simulink model "Junctions7"  (R2020a)
settings: Solver=FixedStepDiscrete  StartTime=0.0  StopTime=0.1  FixedStep=0.1  RelTol=1e-3  EnableMultiTasking=on
settings Model: Creator=BEAR  LastModifiedBy=bzhan
settings SolverCC: AutoInsertRateTranBlk=on
settings DataIOCC: LimitDataPoints=on  ReturnWorkspaceOutputs=off
settings OptimizationCC: LifeSpan=inf
settings DebuggingCC: AllowSymbolicDim=off  SFUnexpectedBacktrackingDiag=warning  SFNoUnconditionalDefaultTransitionDiag=warning  SFExecutionAtInitializationDiag=none  ArithmeticOperatorsInVariantConditions=warning
settings SFSimCC: SimUseLocalCustomCode=off  CustomCodeUndefinedFunction=UseInterfaceOnly
settings RTWCC: RTWUseLocalCustomCode=off
settings CodeAppCC: StateflowObjectComments=on
settings GRTTargetCC: TargetLangStandard=C89/C90 (ANSI)
settings ConfigComp: CovMetricSettings=dw  CovHtmlReporting=on  CovSaveCumulativeToWorkspaceVar=on  CovSaveSingleToWorkspaceVar=on  CovShowResultsExplorer=off  CovExternalEMLEnable=off  CovSFcnEnable=off

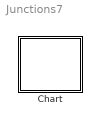
== system Junctions7 ==
  Chart : Stateflow chart  TreatAsAtomicUnit=on

== stateflow chart Junctions7/Chart ==
  state A
    en: f("enA")
    ex: f("exA")
  state C
    en: f("enC")
    ex: f("exC")
  (default) -> A : {x=1;y=2;z=3;}
  A -> (junction 5) [order 1] : [x>2]/{f("xge2")}
  (junction 15) -> C [order 1] : [z>2]/{f("zge2")}
  (junction 5) -> (junction 15) [order 1] : [y>2]/{f("yge2")}
  A -> (junction 5) [order 2] : [x==2]/{f("xeq2")}
  (junction 5) -> (junction 15) [order 2] : [y==2]/{f("yeq2")}
  (junction 15) -> C [order 2] : [z==2]/{f("zeq2")}
  A -> (junction 5) [order 3] : [x<2]/{f("xle2")}
  (junction 15) -> C [order 3] : [z<2]/{f("zle2")}
  (junction 5) -> (junction 15) [order 3] : [y<2]/{f("yle2")}
  data: s function_input; x local; y local; z local
  function f(s):
    | function f(s)
    |     fprintf(s+"\n");
